simulink library "MESSIN_Library"  (R2024a)
settings: Solver=VariableStepAuto  StartTime=0.0  StopTime=10.0  RelTol=1e-3
undefined symbols (not defined in the file or in its folder): actuatorCommand, commandedActuator, commandMode, externCommand, ready, remoteControlDevice, sensor, supervisor, timestampUTC, useXNAllocation
libraries: $bdroot x376, etargetslib x52, simulink x19
(part 5 of 5)

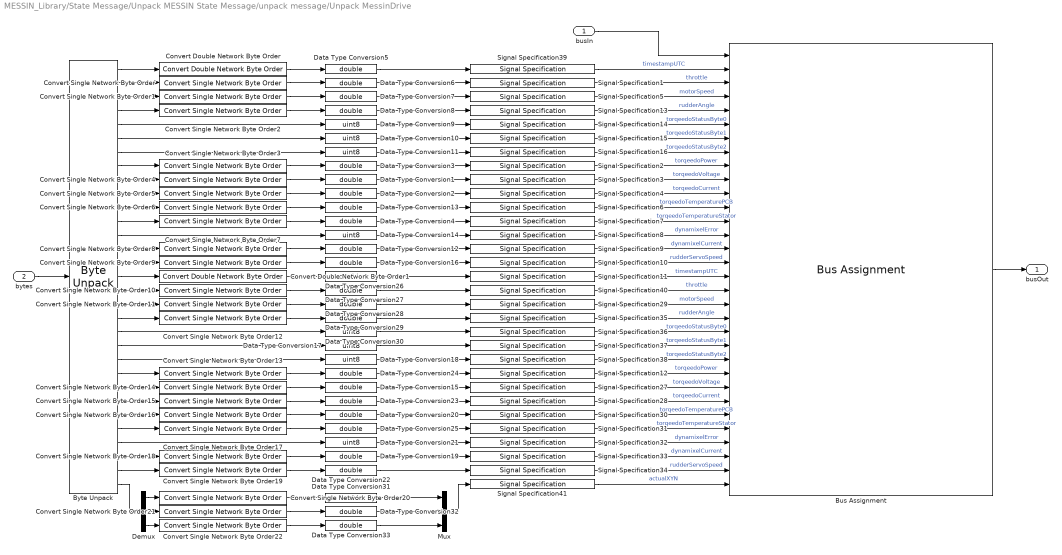
== system MESSIN_Library/State Message/Unpack MESSIN State Message/unpack message/Unpack MessinDrive ==
  busIn : Inport
  bytes : Inport  Port=2
  Bus Assignment : BusAssignment  AssignedSignals=sensor.messinDrive.actuatorStarboard.timestampUTC,sensor.messinDrive.actuatorStarboard.throttle,sensor.messinDrive.actuatorStarboard.motorSpeed,sensor.messinDrive.actuatorStarboard.rudderAngle,sensor.messinDrive.actuatorStarboard.torqeedoStatusByte0,sensor.messinDrive.actuatorStarboard.torqeedoStatusByte1,sensor.messinDrive.actuatorStarboard.torqeedoStatusByte2,sensor.messinDrive.actuatorStarboard.torqeedoPower,sensor.messinDrive.actuatorStarboard.torqeedoVoltage,sensor.messinDrive.actuatorStarboard.torqeedoCurrent,sensor.messinDrive.actuatorStarboard.torqeedoTemperaturePCB,sensor.messinDrive.actuatorStarboard.torqeedoTemperatureStator,sensor.messinDrive.actuatorStarboard.dynamixelError,sensor.messinDrive.actuatorStarboard.dynamixelCurrent,sensor.messinDrive.actuatorStarboard.rudderServoSpeed,sensor.messinDrive.actuatorPortside.timestampUTC,sensor.messinDrive.actuatorPortside.throttle,sensor.messinDrive.actuatorPortside.motorSpeed,sensor.messinDrive.actuatorPortside.rudderAngle,sensor.messinDrive.actuatorPortside.torqeedoStatusByte0,sensor.messinDrive.actuatorPortside.torqeedoStatusByte1,sensor.messinDrive.actuatorPortside.torqeedoStatusByte2,sensor.messinDrive.actuatorPortside.torqeedoPower,sensor.messinDrive.actuatorPortside.torqeedoVoltage,sensor.messinDrive.actuatorPortside.torqeedoCurrent,sensor.messinDrive.actuatorPortside.torqeedoTemperaturePCB,sensor.messinDrive.actuatorPortside.torqeedoTemperatureStator,sensor.messinDrive.actuatorPortside.dynamixelError,sensor.messinDrive.actuatorPortside.dynamixelCurrent,sensor.messinDrive.actuatorPortside.rudderServoSpeed,sensor.messinDrive.actualXYN
  Byte Unpack : etargetslib/Byte Unpack  dimensions={1,1,1,1,1,1,1,1,1,1,1,1,1,1,1,1,1,1,1,1,1,1,1,1,1,1,1,1,1,1,3}  datatypes={'double','single','single','single','uint8','uint8','uint8','single','single','single','single','single','uint8','single','single','double','single','single','single','uint8','uint8','uint8','single','single','single','single','single','uint8','single','single','single'}  byteAlign=1
      settings: LibrarySourceBlock=embeddedtargetslib/Host Communication/Byte Unpack
  Convert Double Network Byte Order : $bdroot/Utilities/Convert Double Network Byte Order
  Convert Double Network Byte Order1 : $bdroot/Utilities/Convert Double Network Byte Order
  Convert Single Network Byte Order{,1..22} (23 alike) : $bdroot/Utilities/Convert Single Network Byte Order
  Data Type Conversion{1..8,12..13,15..16,19..20,22..29,31..33} (25 alike) : DataTypeConversion  OutDataTypeStr=double  SaturateOnIntegerOverflow=off  RndMeth=Floor
  Data Type Conversion{9..11,14,17..18,21,30} (8 alike) : DataTypeConversion  OutDataTypeStr=uint8  SaturateOnIntegerOverflow=off  RndMeth=Floor
  Demux : Demux  Outputs=3
  Mux : Mux  Inputs=3
  Signal Specification1 : SignalSpecification  OutDataTypeStr=double  Unit=1  Dimensions=1
  Signal Specification{5,10,29,34} (4 alike) : SignalSpecification  OutDataTypeStr=double  Unit=rad/s  Dimensions=1
  Signal Specification11 : SignalSpecification  OutDataTypeStr=double  Unit=s  Dimensions=1
  Signal Specification12 : SignalSpecification  OutDataTypeStr=double  Unit=W  Dimensions=1
  Signal Specification13 : SignalSpecification  OutDataTypeStr=double  Unit=rad  Dimensions=1
  Signal Specification{8,14..16,32,36..38} (8 alike) : SignalSpecification  OutDataTypeStr=uint8  Unit=1  Dimensions=1
  Signal Specification2 : SignalSpecification  OutDataTypeStr=double  Unit=W  Dimensions=1
  Signal Specification27 : SignalSpecification  OutDataTypeStr=double  Unit=V  Dimensions=1
  Signal Specification{4,9,28,33} (4 alike) : SignalSpecification  OutDataTypeStr=double  Unit=A  Dimensions=1
  Signal Specification3 : SignalSpecification  OutDataTypeStr=double  Unit=V  Dimensions=1
  Signal Specification{6..7,30..31} (4 alike) : SignalSpecification  OutDataTypeStr=double  Unit=°C  Dimensions=1
  Signal Specification35 : SignalSpecification  OutDataTypeStr=double  Unit=rad  Dimensions=1
  Signal Specification39 : SignalSpecification  OutDataTypeStr=double  Unit=s  Dimensions=1
  Signal Specification40 : SignalSpecification  OutDataTypeStr=double  Unit=1  Dimensions=1
  Signal Specification41 : SignalSpecification  OutDataTypeStr=double  Dimensions=3
  busOut : Outport
  wires:
  Data Type Conversion3/1 -> Signal Specification2/1
  Data Type Conversion1/1 -> Signal Specification3/1
  Data Type Conversion2/1 -> Signal Specification4/1
  Data Type Conversion8/1 -> Signal Specification13/1
  Data Type Conversion7/1 -> Signal Specification5/1
  Data Type Conversion6/1 -> Signal Specification1/1
  Data Type Conversion5/1 -> Signal Specification39/1
  Data Type Conversion11/1 -> Signal Specification16/1
  Data Type Conversion10/1 -> Signal Specification15/1
  Data Type Conversion9/1 -> Signal Specification14/1
  Bus Assignment/1 -> busOut/1
  bytes/1 -> Byte Unpack/1
  busIn/1 -> Bus Assignment/1
  Signal Specification10/1 -> Bus Assignment/16  "rudderServoSpeed"
  Signal Specification29/1 -> Bus Assignment/19  "motorSpeed"
  Signal Specification35/1 -> Bus Assignment/20  "rudderAngle"
  Signal Specification8/1 -> Bus Assignment/14  "dynamixelError"
  Signal Specification6/1 -> Bus Assignment/12  "torqeedoTemperaturePCB"
  Signal Specification3/1 -> Bus Assignment/10  "torqeedoVoltage"
  Signal Specification9/1 -> Bus Assignment/15  "dynamixelCurrent"
  Signal Specification16/1 -> Bus Assignment/8  "torqeedoStatusByte2"
  Signal Specification39/1 -> Bus Assignment/2  "timestampUTC"
  Signal Specification13/1 -> Bus Assignment/5  "rudderAngle"
  Signal Specification33/1 -> Bus Assignment/30  "dynamixelCurrent"
  Signal Specification36/1 -> Bus Assignment/21  "torqeedoStatusByte0"
  Signal Specification1/1 -> Bus Assignment/3  "throttle"
  Signal Specification28/1 -> Bus Assignment/26  "torqeedoCurrent"
  Signal Specification11/1 -> Bus Assignment/17  "timestampUTC"
  Signal Specification27/1 -> Bus Assignment/25  "torqeedoVoltage"
  Signal Specification2/1 -> Bus Assignment/9  "torqeedoPower"
  Signal Specification12/1 -> Bus Assignment/24  "torqeedoPower"
  Signal Specification40/1 -> Bus Assignment/18  "throttle"
  Signal Specification15/1 -> Bus Assignment/7  "torqeedoStatusByte1"
  Signal Specification31/1 -> Bus Assignment/28  "torqeedoTemperatureStator"
  Signal Specification7/1 -> Bus Assignment/13  "torqeedoTemperatureStator"
  Signal Specification37/1 -> Bus Assignment/22  "torqeedoStatusByte1"
  Signal Specification30/1 -> Bus Assignment/27  "torqeedoTemperaturePCB"
  Signal Specification38/1 -> Bus Assignment/23  "torqeedoStatusByte2"
  Signal Specification32/1 -> Bus Assignment/29  "dynamixelError"
  Signal Specification4/1 -> Bus Assignment/11  "torqeedoCurrent"
  Signal Specification14/1 -> Bus Assignment/6  "torqeedoStatusByte0"
  Signal Specification34/1 -> Bus Assignment/31  "rudderServoSpeed"
  Signal Specification5/1 -> Bus Assignment/4  "motorSpeed"
  Signal Specification41/1 -> Bus Assignment/32  "actualXYN"
  Data Type Conversion14/1 -> Signal Specification8/1
  Data Type Conversion4/1 -> Signal Specification7/1
  Data Type Conversion13/1 -> Signal Specification6/1
  Data Type Conversion16/1 -> Signal Specification10/1
  Convert Double Network Byte Order/1 -> Data Type Conversion5/1
  Convert Single Network Byte Order/1 -> Data Type Conversion6/1
  Convert Single Network Byte Order1/1 -> Data Type Conversion7/1
  Convert Single Network Byte Order2/1 -> Data Type Conversion8/1
  Convert Single Network Byte Order3/1 -> Data Type Conversion3/1
  Convert Single Network Byte Order4/1 -> Data Type Conversion1/1
  Convert Single Network Byte Order5/1 -> Data Type Conversion2/1
  Convert Single Network Byte Order6/1 -> Data Type Conversion13/1
  Convert Single Network Byte Order7/1 -> Data Type Conversion4/1
  Convert Single Network Byte Order8/1 -> Data Type Conversion12/1
  Convert Single Network Byte Order9/1 -> Data Type Conversion16/1
  Byte Unpack/1 -> Convert Double Network Byte Order/1
  Byte Unpack/2 -> Convert Single Network Byte Order/1
  Byte Unpack/3 -> Convert Single Network Byte Order1/1
  Byte Unpack/4 -> Convert Single Network Byte Order2/1
  Byte Unpack/5 -> Data Type Conversion9/1
  Byte Unpack/6 -> Data Type Conversion10/1
  Byte Unpack/7 -> Data Type Conversion11/1
  Byte Unpack/8 -> Convert Single Network Byte Order3/1
  Byte Unpack/9 -> Convert Single Network Byte Order4/1
  Byte Unpack/10 -> Convert Single Network Byte Order5/1
  Byte Unpack/11 -> Convert Single Network Byte Order6/1
  Byte Unpack/12 -> Convert Single Network Byte Order7/1
  Byte Unpack/13 -> Data Type Conversion14/1
  Byte Unpack/15 -> Convert Single Network Byte Order9/1
  Data Type Conversion12/1 -> Signal Specification9/1
  Byte Unpack/14 -> Convert Single Network Byte Order8/1
  Byte Unpack/29 -> Convert Single Network Byte Order18/1
  Data Type Conversion19/1 -> Signal Specification33/1
  Byte Unpack/30 -> Convert Single Network Byte Order19/1
  Byte Unpack/28 -> Data Type Conversion21/1
  Byte Unpack/27 -> Convert Single Network Byte Order17/1
  Byte Unpack/26 -> Convert Single Network Byte Order16/1
  Byte Unpack/25 -> Convert Single Network Byte Order15/1
  Byte Unpack/24 -> Convert Single Network Byte Order14/1
  Byte Unpack/23 -> Convert Single Network Byte Order13/1
  Byte Unpack/22 -> Data Type Conversion18/1
  Byte Unpack/21 -> Data Type Conversion17/1
  Byte Unpack/20 -> Data Type Conversion30/1
  Byte Unpack/19 -> Convert Single Network Byte Order12/1
  Byte Unpack/18 -> Convert Single Network Byte Order11/1
  Byte Unpack/17 -> Convert Single Network Byte Order10/1
  Byte Unpack/16 -> Convert Double Network Byte Order1/1
  Convert Single Network Byte Order19/1 -> Data Type Conversion22/1
  Convert Single Network Byte Order18/1 -> Data Type Conversion19/1
  Convert Single Network Byte Order17/1 -> Data Type Conversion25/1
  Convert Single Network Byte Order16/1 -> Data Type Conversion20/1
  Convert Single Network Byte Order15/1 -> Data Type Conversion23/1
  Convert Single Network Byte Order14/1 -> Data Type Conversion15/1
  Convert Single Network Byte Order13/1 -> Data Type Conversion24/1
  Convert Single Network Byte Order12/1 -> Data Type Conversion29/1
  Convert Single Network Byte Order11/1 -> Data Type Conversion28/1
  Convert Single Network Byte Order10/1 -> Data Type Conversion27/1
  Convert Double Network Byte Order1/1 -> Data Type Conversion26/1
  Data Type Conversion22/1 -> Signal Specification34/1
  Data Type Conversion20/1 -> Signal Specification30/1
  Data Type Conversion25/1 -> Signal Specification31/1
  Data Type Conversion21/1 -> Signal Specification32/1
  Data Type Conversion30/1 -> Signal Specification36/1
  Data Type Conversion17/1 -> Signal Specification37/1
  Data Type Conversion18/1 -> Signal Specification38/1
  Data Type Conversion26/1 -> Signal Specification11/1
  Data Type Conversion27/1 -> Signal Specification40/1
  Data Type Conversion28/1 -> Signal Specification29/1
  Data Type Conversion29/1 -> Signal Specification35/1
  Data Type Conversion23/1 -> Signal Specification28/1
  Data Type Conversion15/1 -> Signal Specification27/1
  Data Type Conversion24/1 -> Signal Specification12/1
  Byte Unpack/31 -> Demux/1
  Demux/1 -> Convert Single Network Byte Order20/1
  Demux/2 -> Convert Single Network Byte Order21/1
  Demux/3 -> Convert Single Network Byte Order22/1
  Convert Single Network Byte Order20/1 -> Data Type Conversion31/1
  Convert Single Network Byte Order21/1 -> Data Type Conversion32/1
  Convert Single Network Byte Order22/1 -> Data Type Conversion33/1
  Data Type Conversion33/1 -> Mux/3
  Data Type Conversion32/1 -> Mux/2
  Data Type Conversion31/1 -> Mux/1
  Mux/1 -> Signal Specification41/1

== system MESSIN_Library/State Message/Unpack MESSIN State Message/unpack message/Unpack RCD ==
  busIn : Inport
  bytes : Inport  Port=2
  Bus Assignment : BusAssignment  AssignedSignals=remoteControlDevice.timestampUTC,remoteControlDevice.joystickLeft,remoteControlDevice.joystickRight
  Byte Unpack : etargetslib/Byte Unpack  dimensions={1,3,3}  datatypes={'double','single','single'}  byteAlign=1
      settings: LibrarySourceBlock=embeddedtargetslib/Host Communication/Byte Unpack
  Convert Double Network Byte Order : $bdroot/Utilities/Convert Double Network Byte Order
  Convert Single Network Byte Order{,1..5} (6 alike) : $bdroot/Utilities/Convert Single Network Byte Order
  Data Type Conversion{,1..6} (7 alike) : DataTypeConversion  OutDataTypeStr=double  SaturateOnIntegerOverflow=off  RndMeth=Floor
  Demux : Demux  Outputs=3
  Demux1 : Demux  Outputs=3
  Mux : Mux  Inputs=3
  Mux1 : Mux  Inputs=3
  Signal Specification15 : SignalSpecification  OutDataTypeStr=double  Unit=s  Dimensions=1
  Signal Specification16 : SignalSpecification  OutDataTypeStr=double  Unit=1  Dimensions=3
  Signal Specification17 : SignalSpecification  OutDataTypeStr=double  Unit=1  Dimensions=3
  busOut : Outport
  wires:
  Bus Assignment/1 -> busOut/1
  bytes/1 -> Byte Unpack/1
  busIn/1 -> Bus Assignment/1
  Convert Double Network Byte Order/1 -> Data Type Conversion/1
  Convert Single Network Byte Order/1 -> Data Type Conversion3/1
  Convert Single Network Byte Order1/1 -> Data Type Conversion4/1
  Convert Single Network Byte Order2/1 -> Data Type Conversion5/1
  Signal Specification15/1 -> Bus Assignment/2  "timestampUTC"
  Signal Specification17/1 -> Bus Assignment/4  "joystickRight"
  Signal Specification16/1 -> Bus Assignment/3  "joystickLeft"
  Data Type Conversion/1 -> Signal Specification15/1
  Data Type Conversion5/1 -> Mux/3
  Data Type Conversion4/1 -> Mux/2
  Data Type Conversion3/1 -> Mux/1
  Demux/1 -> Convert Single Network Byte Order/1
  Demux/2 -> Convert Single Network Byte Order1/1
  Demux/3 -> Convert Single Network Byte Order2/1
  Demux1/3 -> Convert Single Network Byte Order5/1
  Demux1/2 -> Convert Single Network Byte Order4/1
  Demux1/1 -> Convert Single Network Byte Order3/1
  Data Type Conversion1/1 -> Mux1/1
  Data Type Conversion2/1 -> Mux1/2
  Data Type Conversion6/1 -> Mux1/3
  Convert Single Network Byte Order5/1 -> Data Type Conversion6/1
  Convert Single Network Byte Order4/1 -> Data Type Conversion2/1
  Convert Single Network Byte Order3/1 -> Data Type Conversion1/1
  Mux/1 -> Signal Specification16/1
  Mux1/1 -> Signal Specification17/1
  Byte Unpack/2 -> Demux/1
  Byte Unpack/1 -> Convert Double Network Byte Order/1
  Byte Unpack/3 -> Demux1/1

== system MESSIN_Library/State Message/Unpack MESSIN State Message/unpack message/Unpack Supervisor ==
  busIn : Inport
  bytes : Inport  Port=2
  Bus Assignment : BusAssignment  AssignedSignals=supervisor.torqeedoPoweredOn,supervisor.actuatorsEnabled,supervisor.lightEnabled,supervisor.actuatorsSynchronized,supervisor.externModeEnabled,supervisor.internalOperationMode
  Byte Unpack : etargetslib/Byte Unpack  dimensions={1,1}  datatypes={'uint8','uint8'}  byteAlign=1
      settings: LibrarySourceBlock=embeddedtargetslib/Host Communication/Byte Unpack
  Data Type Conversion1 : DataTypeConversion  OutDataTypeStr=uint8  SaturateOnIntegerOverflow=off  RndMeth=Floor
  Data Type Conversion2 : DataTypeConversion  OutDataTypeStr=boolean  SaturateOnIntegerOverflow=off  RndMeth=Floor
  Demux : Demux  Outputs=8
  Selector : Selector  InputPortWidth=8  IndexOptions=Index vector (dialog)  Indices=[8 7 6 5 4 3 2 1]  OutputSizes=1
  Signal Specification{1..5} (5 alike) : SignalSpecification  OutDataTypeStr=boolean  Unit=1  Dimensions=1
  Signal Specification6 : SignalSpecification  OutDataTypeStr=uint8  Unit=1  Dimensions=1
  Terminator : Terminator
  Terminator1 : Terminator
  Terminator2 : Terminator
  Unpack Bitfield : $bdroot/Utilities/Unpack Bitfield
  busOut : Outport
  wires:
  busIn/1 -> Bus Assignment/1
  bytes/1 -> Byte Unpack/1
  Bus Assignment/1 -> busOut/1
  Signal Specification3/1 -> Bus Assignment/4  "lightEnabled"
  Signal Specification1/1 -> Bus Assignment/2  "torqeedoPoweredOn"
  Signal Specification2/1 -> Bus Assignment/3  "actuatorsEnabled"
  Signal Specification6/1 -> Bus Assignment/7  "internalOperationMode"
  Signal Specification4/1 -> Bus Assignment/5  "actuatorsSynchronized"
  Signal Specification5/1 -> Bus Assignment/6  "externModeEnabled"
  Unpack Bitfield/1 -> Data Type Conversion2/1
  Data Type Conversion2/1 -> Selector/1
  Demux/1 -> Signal Specification1/1
  Demux/2 -> Signal Specification2/1
  Demux/3 -> Signal Specification3/1
  Demux/4 -> Signal Specification4/1
  Demux/5 -> Signal Specification5/1
  Demux/6 -> Terminator/1
  Demux/7 -> Terminator1/1
  Demux/8 -> Terminator2/1
  Selector/1 -> Demux/1
  Data Type Conversion1/1 -> Signal Specification6/1
  Byte Unpack/2 -> Data Type Conversion1/1
  Byte Unpack/1 -> Unpack Bitfield/1

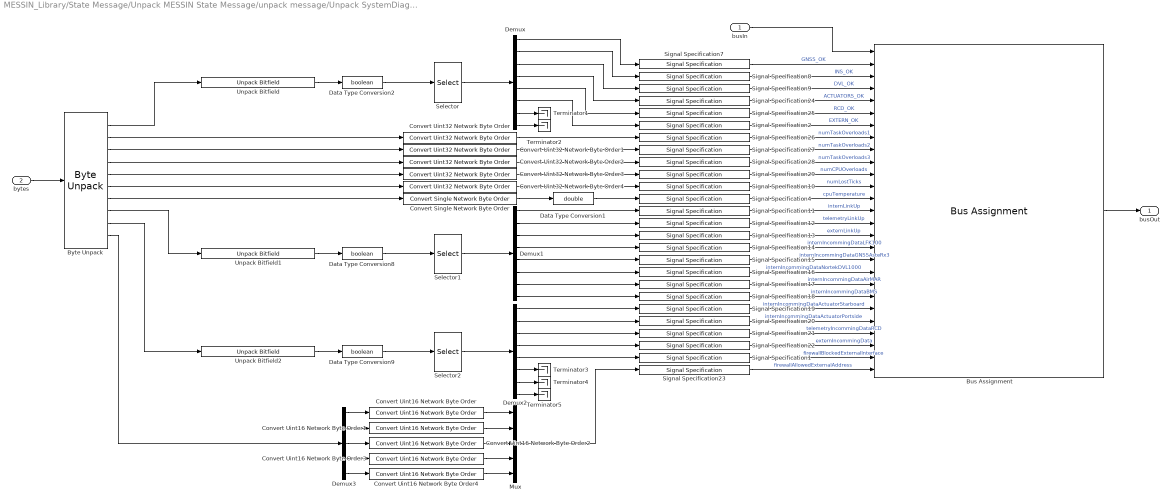
== system MESSIN_Library/State Message/Unpack MESSIN State Message/unpack message/Unpack SystemDiagnostics ==
  busIn : Inport
  bytes : Inport  Port=2
  Bus Assignment : BusAssignment  AssignedSignals=systemDiagnostics.GNSS_OK,systemDiagnostics.INS_OK,systemDiagnostics.DVL_OK,systemDiagnostics.ACTUATORS_OK,systemDiagnostics.RCD_OK,systemDiagnostics.EXTERN_OK,systemDiagnostics.details.hardware.numTaskOverloads1,systemDiagnostics.details.hardware.numTaskOverloads2,systemDiagnostics.details.hardware.numTaskOverloads3,systemDiagnostics.details.hardware.numCPUOverloads,systemDiagnostics.details.hardware.numLostTicks,systemDiagnostics.details.hardware.cpuTemperature,systemDiagnostics.details.network.internLinkUp,systemDiagnostics.details.network.telemetryLinkUp,systemDiagnostics.details.network.externLinkUp,systemDiagnostics.details.network.internIncommingDataLFK100,systemDiagnostics.details.network.internIncommingDataGNSSAsteRx3,systemDiagnostics.details.network.internIncommingDataNortekDVL1000,systemDiagnostics.details.network.internIncommingDataAirMAR,systemDiagnostics.details.network.internIncommingDataBMS,systemDiagnostics.details.network.internIncommingDataActuatorStarboard,systemDiagnostics.details.network.internIncommingDataActuatorPortside,systemDiagnostics.details.network.telemetryIncommingDataRCD,systemDiagnostics.details.network.externIncommingData,systemDiagnostics.details.network.firewallBlockedExternalInterface,systemDiagnostics.details.network.firewallAllowedExternalAddress
  Byte Unpack : etargetslib/Byte Unpack  dimensions={1,1,1,1,1,1,1,1,1,5}  datatypes={'uint8','uint32','uint32','uint32','uint32','uint32','single','uint8','uint8','uint16'}  byteAlign=1
      settings: LibrarySourceBlock=embeddedtargetslib/Host Communication/Byte Unpack
  Convert Single Network Byte Order : $bdroot/Utilities/Convert Single Network Byte Order
  Convert Uint16 Network Byte Order{,1..4} (5 alike) : $bdroot/Utilities/Convert Uint16 Network Byte Order
  Convert Uint32 Network Byte Order{,1..4} (5 alike) : $bdroot/Utilities/Convert Uint32 Network Byte Order
  Data Type Conversion1 : DataTypeConversion  OutDataTypeStr=double  SaturateOnIntegerOverflow=off  RndMeth=Floor
  Data Type Conversion2 : DataTypeConversion  OutDataTypeStr=boolean  SaturateOnIntegerOverflow=off  RndMeth=Floor
  Data Type Conversion8 : DataTypeConversion  OutDataTypeStr=boolean  SaturateOnIntegerOverflow=off  RndMeth=Floor
  Data Type Conversion9 : DataTypeConversion  OutDataTypeStr=boolean  SaturateOnIntegerOverflow=off  RndMeth=Floor
  Demux : Demux  Outputs=8
  Demux1 : Demux  Outputs=8
  Demux2 : Demux  Outputs=8
  Demux3 : Demux  Outputs=5
  Mux : Mux  Inputs=5
  Selector : Selector  InputPortWidth=8  IndexOptions=Index vector (dialog)  Indices=[8 7 6 5 4 3 2 1]  OutputSizes=1
  Selector1 : Selector  InputPortWidth=8  IndexOptions=Index vector (dialog)  Indices=[8 7 6 5 4 3 2 1]  OutputSizes=1
  Selector2 : Selector  InputPortWidth=8  IndexOptions=Index vector (dialog)  Indices=[8 7 6 5 4 3 2 1]  OutputSizes=1
  Signal Specification{1..2,7..9,11..22,24..25} (19 alike) : SignalSpecification  OutDataTypeStr=boolean  Unit=1  Dimensions=1
  Signal Specification{10,26..29} (5 alike) : SignalSpecification  OutDataTypeStr=uint32  Unit=1  Dimensions=1
  Signal Specification23 : SignalSpecification  OutDataTypeStr=uint16  Unit=1  Dimensions=5
  Signal Specification4 : SignalSpecification  OutDataTypeStr=double  Unit=°C  Dimensions=1
  Terminator{1..5} (5 alike) : Terminator
  Unpack Bitfield : $bdroot/Utilities/Unpack Bitfield
  Unpack Bitfield1 : $bdroot/Utilities/Unpack Bitfield
  Unpack Bitfield2 : $bdroot/Utilities/Unpack Bitfield
  busOut : Outport
  wires:
  Byte Unpack/1 -> Unpack Bitfield/1
  Selector/1 -> Demux/1
  Demux/8 -> Terminator2/1
  Demux/7 -> Terminator1/1
  Demux/5 -> Signal Specification25/1
  Demux/4 -> Signal Specification24/1
  Demux/3 -> Signal Specification9/1
  Demux/2 -> Signal Specification8/1
  Demux/1 -> Signal Specification7/1
  Data Type Conversion2/1 -> Selector/1
  Unpack Bitfield/1 -> Data Type Conversion2/1
  Bus Assignment/1 -> busOut/1
  bytes/1 -> Byte Unpack/1
  busIn/1 -> Bus Assignment/1
  Signal Specification10/1 -> Bus Assignment/12  "numLostTicks"
  Signal Specification29/1 -> Bus Assignment/11  "numCPUOverloads"
  Signal Specification11/1 -> Bus Assignment/14  "internLinkUp"
  Signal Specification26/1 -> Bus Assignment/8  "numTaskOverloads1"
  Signal Specification27/1 -> Bus Assignment/9  "numTaskOverloads2"
  Signal Specification28/1 -> Bus Assignment/10  "numTaskOverloads3"
  Convert Uint32 Network Byte Order/1 -> Signal Specification26/1
  Convert Uint32 Network Byte Order1/1 -> Signal Specification27/1
  Convert Uint32 Network Byte Order2/1 -> Signal Specification28/1
  Convert Uint32 Network Byte Order3/1 -> Signal Specification29/1
  Convert Uint32 Network Byte Order4/1 -> Signal Specification10/1
  Unpack Bitfield1/1 -> Data Type Conversion8/1
  Data Type Conversion8/1 -> Selector1/1
  Selector1/1 -> Demux1/1
  Demux1/1 -> Signal Specification11/1
  Demux1/2 -> Signal Specification12/1
  Demux1/3 -> Signal Specification13/1
  Demux1/4 -> Signal Specification14/1
  Demux1/5 -> Signal Specification15/1
  Demux1/6 -> Signal Specification16/1
  Demux1/7 -> Signal Specification17/1
  Demux1/8 -> Signal Specification18/1
  Unpack Bitfield2/1 -> Data Type Conversion9/1
  Data Type Conversion9/1 -> Selector2/1
  Demux2/6 -> Terminator3/1
  Demux2/7 -> Terminator4/1
  Demux2/8 -> Terminator5/1
  Selector2/1 -> Demux2/1
  Demux2/1 -> Signal Specification19/1
  Demux2/2 -> Signal Specification20/1
  Demux2/3 -> Signal Specification21/1
  Demux2/4 -> Signal Specification22/1
  Demux2/5 -> Signal Specification1/1
  Demux3/5 -> Convert Uint16 Network Byte Order4/1
  Demux3/4 -> Convert Uint16 Network Byte Order3/1
  Demux3/3 -> Convert Uint16 Network Byte Order2/1
  Demux3/2 -> Convert Uint16 Network Byte Order1/1
  Demux3/1 -> Convert Uint16 Network Byte Order/1
  Convert Uint16 Network Byte Order/1 -> Mux/1
  Convert Uint16 Network Byte Order1/1 -> Mux/2
  Convert Uint16 Network Byte Order2/1 -> Mux/3
  Convert Uint16 Network Byte Order3/1 -> Mux/4
  Convert Uint16 Network Byte Order4/1 -> Mux/5
  Mux/1 -> Signal Specification23/1
  Signal Specification23/1 -> Bus Assignment/27  "firewallAllowedExternalAddress"
  Signal Specification12/1 -> Bus Assignment/15  "telemetryLinkUp"
  Signal Specification13/1 -> Bus Assignment/16  "externLinkUp"
  Signal Specification14/1 -> Bus Assignment/17  "internIncommingDataLFK100"
  Signal Specification15/1 -> Bus Assignment/18  "internIncommingDataGNSSAsteRx3"
  Signal Specification16/1 -> Bus Assignment/19  "internIncommingDataNortekDVL1000"
  Signal Specification17/1 -> Bus Assignment/20  "internIncommingDataAirMAR"
  Signal Specification18/1 -> Bus Assignment/21  "internIncommingDataBMS"
  Signal Specification19/1 -> Bus Assignment/22  "internIncommingDataActuatorStarboard"
  Signal Specification20/1 -> Bus Assignment/23  "internIncommingDataActuatorPortside"
  Signal Specification21/1 -> Bus Assignment/24  "telemetryIncommingDataRCD"
  Signal Specification22/1 -> Bus Assignment/25  "externIncommingData"
  Signal Specification1/1 -> Bus Assignment/26  "firewallBlockedExternalInterface"
  Demux/6 -> Signal Specification2/1
  Signal Specification2/1 -> Bus Assignment/7  "EXTERN_OK"
  Signal Specification25/1 -> Bus Assignment/6  "RCD_OK"
  Signal Specification24/1 -> Bus Assignment/5  "ACTUATORS_OK"
  Signal Specification9/1 -> Bus Assignment/4  "DVL_OK"
  Signal Specification8/1 -> Bus Assignment/3  "INS_OK"
  Signal Specification7/1 -> Bus Assignment/2  "GNSS_OK"
  Byte Unpack/2 -> Convert Uint32 Network Byte Order/1
  Byte Unpack/3 -> Convert Uint32 Network Byte Order1/1
  Byte Unpack/4 -> Convert Uint32 Network Byte Order2/1
  Byte Unpack/5 -> Convert Uint32 Network Byte Order3/1
  Byte Unpack/6 -> Convert Uint32 Network Byte Order4/1
  Byte Unpack/7 -> Convert Single Network Byte Order/1
  Convert Single Network Byte Order/1 -> Data Type Conversion1/1
  Data Type Conversion1/1 -> Signal Specification4/1
  Signal Specification4/1 -> Bus Assignment/13  "cpuTemperature"
  Byte Unpack/8 -> Unpack Bitfield1/1
  Byte Unpack/9 -> Unpack Bitfield2/1
  Byte Unpack/10 -> Demux3/1

== system MESSIN_Library/State Message/Unpack MESSIN State Message/unpack message/Unpack INS/Subsystem ==
  byte : Inport
  Data Type Conversion8 : DataTypeConversion  OutDataTypeStr=boolean  SaturateOnIntegerOverflow=off  RndMeth=Floor
  Demux1 : Demux  Outputs=8
  Selector1 : Selector  InputPortWidth=8  IndexOptions=Index vector (dialog)  Indices=[8 7 6 5 4 3 2 1]  OutputSizes=1
  Terminator{,1..5} (6 alike) : Terminator
  Unpack Bitfield : $bdroot/Utilities/Unpack Bitfield
  bit0 : Outport
  bit1 : Outport  Port=2
  wires:
  Demux1/7 -> Terminator4/1
  Unpack Bitfield/1 -> Data Type Conversion8/1
  Demux1/1 -> bit0/1
  Demux1/3 -> Terminator/1
  Demux1/4 -> Terminator1/1
  Demux1/6 -> Terminator3/1
  Data Type Conversion8/1 -> Selector1/1
  Demux1/8 -> Terminator5/1
  Selector1/1 -> Demux1/1
  Demux1/5 -> Terminator2/1
  Demux1/2 -> bit1/1
  byte/1 -> Unpack Bitfield/1

== matlab function MESSIN_Library/Utilities/Make Finite/ReplaceNonfiniteByZeros ==
  data: u input; y output
function y = ReplaceNonfinteByZeros(u)
    y = u;
    y(~isfinite(y)) = 0.0;
end
